simulink model "sf_test"  (R2020a)
settings: Solver=FixedStepDiscrete  StartTime=0.0  StopTime=10.0  RelTol=1e-3
settings Model: Creator=김진성  LastModifiedBy=노호진
settings OptimizationCC: DefaultParameterBehavior=Inlined  EnhancedBackFolding=on  PassReuseOutputArgsAs=Individual arguments  OptimizeBlockOrder=speed  DifferentSizesBufferReuse=on  OptimizationCustomize=off  EfficientTunableParamExpr=on
settings DebuggingCC: ParameterTunabilityLossMsg=error
settings HardwareCC: ProdBitPerPointer=32  ProdBitPerSizeT=32  ProdBitPerPtrDiffT=32  ProdLargestAtomicInteger=Long  ProdLargestAtomicFloat=Double  ProdWordSize=32  ProdHWDeviceType=ARM Compatible->ARM Cortex
settings SFSimCC: MATLABDynamicMemAlloc=off
settings RTWCC: SystemTargetFile=ert.tlc  GenCodeOnly=on  TemplateMakefile=ert_default_tmf  GenerateReport=on  IncludeHyperlinkInReport=on  LaunchReport=on  GenerateTraceInfo=on  GenerateTraceReport=on  GenerateTraceReportSl=on  GenerateTraceReportSf=on  GenerateTraceReportEml=on  GenerateCodeMetricsReport=on  GenerateCodeReplacementReport=on
settings CodeAppCC: ForceParamTrailComments=on  IgnoreCustomStorageClasses=off  OperatorAnnotations=on  SimulinkDataObjDesc=on  SFDataObjDesc=on  InsertBlockDesc=on  StateflowObjectComments=on
settings ERTTargetCC: TargetLangStandard=C99 (ISO)  GenerateSampleERTMain=on  MultiInstanceERTCode=on  CodeInterfacePackaging=Reusable function  InlinedParameterPlacement=NonHierarchical  ERTCustomFileTemplate=example_file_process.tlc

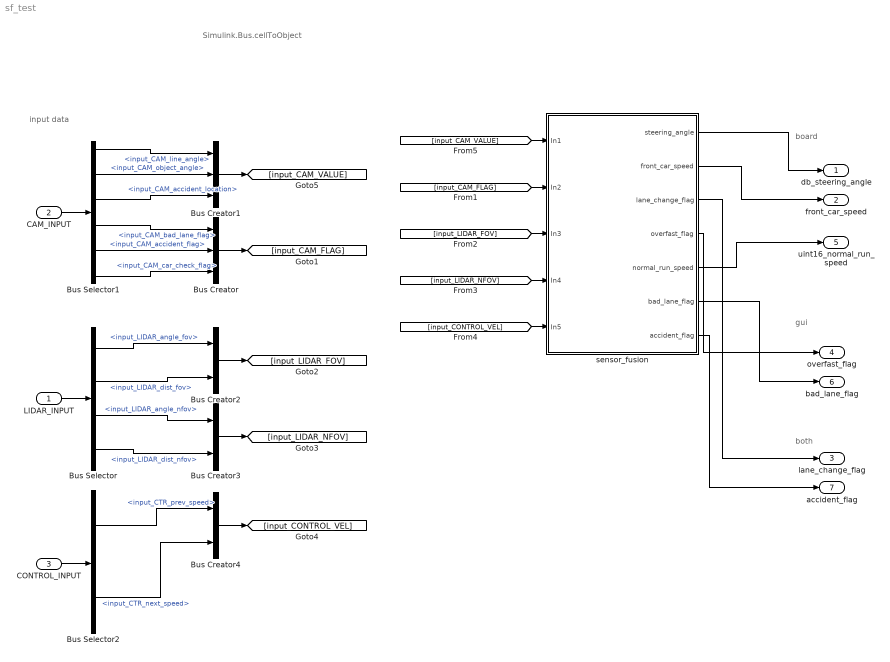
== system sf_test ==
  note: Simulink.Bus.cellToObject
  note: both
  note: gui
  note: board
  note: input data
  LIDAR_INPUT : Inport  OutDataTypeStr=Bus: LIDAR
  CAM_INPUT : Inport  Port=2  OutDataTypeStr=Bus: CAM
  CONTROL_INPUT : Inport  Port=3  OutDataTypeStr=Bus: CONTROL
  Bus Creator : BusCreator  Inputs=3
  Bus Creator1 : BusCreator  Inputs=3
  Bus Creator2 : BusCreator  Inputs=2
  Bus Creator3 : BusCreator  Inputs=2
  Bus Creator4 : BusCreator  Inputs=2
  Bus Selector : BusSelector  OutputSignals=input_LIDAR_angle_fov,input_LIDAR_dist_fov,input_LIDAR_angle_nfov,input_LIDAR_dist_nfov
  Bus Selector1 : BusSelector  OutputSignals=input_CAM_line_angle,input_CAM_object_angle,input_CAM_accident_location,input_CAM_bad_lane_flag,input_CAM_accident_flag,input_CAM_car_check_flag
  Bus Selector2 : BusSelector  OutputSignals=input_CTR_prev_speed,input_CTR_next_speed
  sensor_fusion : Subsystem  TreatAsAtomicUnit=on
      settings: RTWSystemCode=Nonreusable function  RTWFcnNameOpts=Use subsystem name
  db_steering_angle : Outport
  front_car_speed : Outport  Port=2
  lane_change_flag : Outport  Port=3
  overfast_flag : Outport  Port=4
  uint16_normal_run_speed : Outport  Port=5  OutDataTypeStr=uint16
  bad_lane_flag : Outport  Port=6
  accident_flag : Outport  Port=7
  wires:
  sensor_fusion/1(steering_angle) -> db_steering_angle/1
  sensor_fusion/3(lane_change_flag) -> lane_change_flag/1
  sensor_fusion/4(overfast_flag) -> overfast_flag/1
  sensor_fusion/5(normal_run_speed) -> uint16_normal_run_speed/1
  sensor_fusion/2(front_car_speed) -> front_car_speed/1
  sensor_fusion/6(bad_lane_flag) -> bad_lane_flag/1
  sensor_fusion/7(accident_flag) -> accident_flag/1
  LIDAR_INPUT/1 -> Bus Selector/1
  CAM_INPUT/1 -> Bus Selector1/1
  CONTROL_INPUT/1 -> Bus Selector2/1
  Bus Selector1/1 -> Bus Creator1/1  "<input_CAM_line_angle>"
  Bus Selector1/2 -> Bus Creator1/2  "<input_CAM_object_angle>"
  Bus Selector1/3 -> Bus Creator1/3  "<input_CAM_accident_location>"
  Bus Selector1/4 -> Bus Creator/1  "<input_CAM_bad_lane_flag>"
  Bus Selector1/5 -> Bus Creator/2  "<input_CAM_accident_flag>"
  Bus Selector1/6 -> Bus Creator/3  "<input_CAM_car_check_flag>"
  Bus Creator/1 -> [input_CAM_FLAG]
  Bus Creator1/1 -> [input_CAM_VALUE]
  Bus Selector/1 -> Bus Creator2/1  "<input_LIDAR_angle_fov>"
  Bus Selector/2 -> Bus Creator2/2  "<input_LIDAR_dist_fov>"
  Bus Selector/3 -> Bus Creator3/1  "<input_LIDAR_angle_nfov>"
  Bus Selector/4 -> Bus Creator3/2  "<input_LIDAR_dist_nfov>"
  Bus Creator2/1 -> [input_LIDAR_FOV]
  Bus Creator3/1 -> [input_LIDAR_NFOV]
  Bus Selector2/1 -> Bus Creator4/1  "<input_CTR_prev_speed>"
  Bus Selector2/2 -> Bus Creator4/2  "<input_CTR_next_speed>"
  Bus Creator4/1 -> [input_CONTROL_VEL]
  [input_CAM_VALUE] -> sensor_fusion/1(In1)
  [input_CAM_FLAG] -> sensor_fusion/2(In2)
  [input_LIDAR_FOV] -> sensor_fusion/3(In3)
  [input_LIDAR_NFOV] -> sensor_fusion/4(In4)
  [input_CONTROL_VEL] -> sensor_fusion/5(In5)

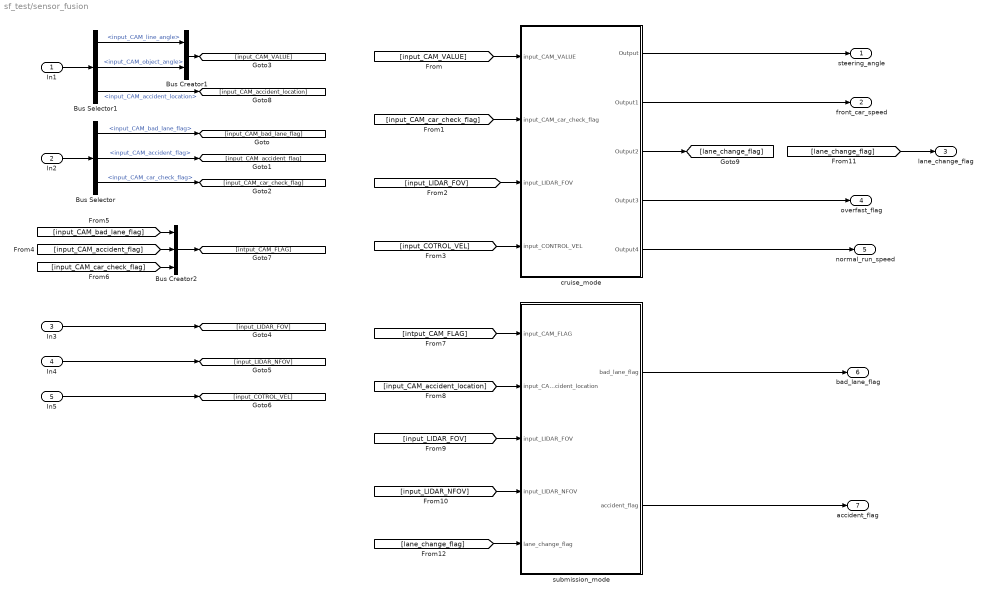
== system sf_test/sensor_fusion ==
  In1 : Inport
  In2 : Inport  Port=2
  In3 : Inport  Port=3
  In4 : Inport  Port=4
  In5 : Inport  Port=5
  Bus Creator1 : BusCreator  Inputs=2
  Bus Creator2 : BusCreator  Inputs=3
  Bus Selector : BusSelector  OutputSignals=input_CAM_bad_lane_flag,input_CAM_accident_flag,input_CAM_car_check_flag
  Bus Selector1 : BusSelector  OutputSignals=input_CAM_line_angle,input_CAM_object_angle,input_CAM_accident_location
  cruise_mode : Subsystem  TreatAsAtomicUnit=on
      settings: RTWSystemCode=Nonreusable function  RTWFcnNameOpts=Use subsystem name
  submission_mode : Subsystem  TreatAsAtomicUnit=on
      settings: RTWSystemCode=Nonreusable function  RTWFcnNameOpts=Use subsystem name
  steering_angle : Outport
  front_car_speed : Outport  Port=2
  lane_change_flag : Outport  Port=3
  overfast_flag : Outport  Port=4
  normal_run_speed : Outport  Port=5  OutDataTypeStr=uint16
  bad_lane_flag : Outport  Port=6
  accident_flag : Outport  Port=7
  wires:
  cruise_mode/1(Output) -> steering_angle/1
  cruise_mode/2(Output1) -> front_car_speed/1
  cruise_mode/4(Output3) -> overfast_flag/1
  cruise_mode/5(Output4) -> normal_run_speed/1
  submission_mode/1(bad_lane_flag) -> bad_lane_flag/1
  submission_mode/2(accident_flag) -> accident_flag/1
  Bus Selector/1 -> [input_CAM_bad_lane_flag]  "<input_CAM_bad_lane_flag>"
  Bus Selector/2 -> [input_CAM_accident_flag]  "<input_CAM_accident_flag>"
  Bus Selector/3 -> [input_CAM_car_check_flag]  "<input_CAM_car_check_flag>"
  In3/1 -> [input_LIDAR_FOV]
  In4/1 -> [input_LIDAR_NFOV]
  In5/1 -> [input_COTROL_VEL]
  [input_CAM_VALUE] -> cruise_mode/1(input_CAM_VALUE)
  [input_CAM_car_check_flag] -> cruise_mode/2(input_CAM_car_check_flag)
  [input_LIDAR_FOV] -> cruise_mode/3(input_LIDAR_FOV)
  [input_COTROL_VEL] -> cruise_mode/4(input_CONTROL_VEL)
  Bus Creator2/1 -> [intput_CAM_FLAG]
  [intput_CAM_FLAG] -> submission_mode/1(input_CAM_FLAG)
  In1/1 -> Bus Selector1/1
  Bus Selector1/1 -> Bus Creator1/1  "<input_CAM_line_angle>"
  Bus Selector1/2 -> Bus Creator1/2  "<input_CAM_object_angle>"
  Bus Selector1/3 -> [input_CAM_accident_location]  "<input_CAM_accident_location>"
  [input_CAM_accident_location] -> submission_mode/2(input_CAM_accident_location)
  [input_LIDAR_FOV] -> submission_mode/3(input_LIDAR_FOV)
  [input_LIDAR_NFOV] -> submission_mode/4(input_LIDAR_NFOV)
  Bus Creator1/1 -> [input_CAM_VALUE]
  [input_CAM_bad_lane_flag] -> Bus Creator2/1
  [input_CAM_accident_flag] -> Bus Creator2/2
  [input_CAM_car_check_flag] -> Bus Creator2/3
  In2/1 -> Bus Selector/1
  cruise_mode/3(Output2) -> [lane_change_flag]
  [lane_change_flag] -> lane_change_flag/1
  [lane_change_flag] -> submission_mode/5(lane_change_flag)

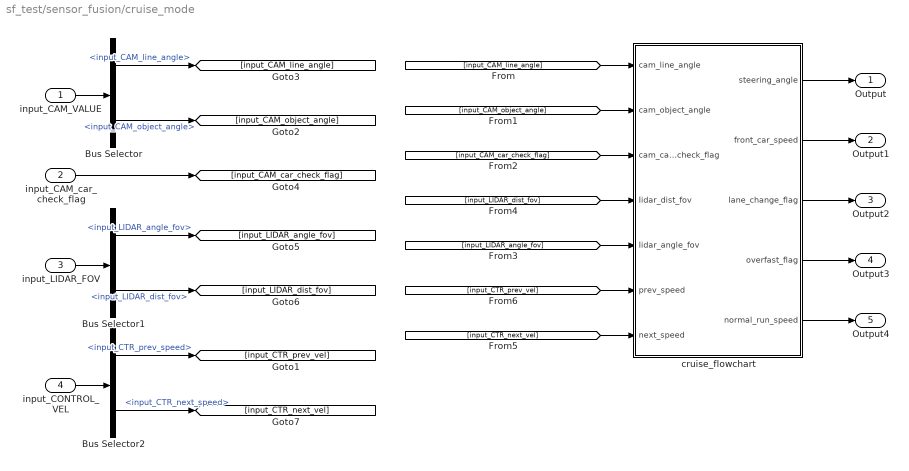
== system sf_test/sensor_fusion/cruise_mode ==
  input_CAM_VALUE : Inport
  input_CAM_car_check_flag : Inport  Port=2
  input_LIDAR_FOV : Inport  Port=3
  input_CONTROL_VEL : Inport  Port=4
  Bus Selector : BusSelector  OutputSignals=input_CAM_line_angle,input_CAM_object_angle
  Bus Selector1 : BusSelector  OutputSignals=input_LIDAR_angle_fov,input_LIDAR_dist_fov
  Bus Selector2 : BusSelector  OutputSignals=input_CTR_prev_speed,input_CTR_next_speed
  cruise_flowchart : Stateflow chart  TreatAsAtomicUnit=on
      settings: RTWSystemCode=Nonreusable function  RTWFcnNameOpts=Use subsystem name
  Output : Outport
  Output1 : Outport  Port=2
  Output2 : Outport  Port=3
  Output3 : Outport  Port=4
  Output4 : Outport  Port=5
  wires:
  [input_CAM_line_angle] -> cruise_flowchart/1(cam_line_angle)
  [input_CAM_object_angle] -> cruise_flowchart/2(cam_object_angle)
  [input_CAM_car_check_flag] -> cruise_flowchart/3(cam_car_check_flag)
  [input_LIDAR_angle_fov] -> cruise_flowchart/5(Iidar_angle_fov)
  cruise_flowchart/1(steering_angle) -> Output/1
  cruise_flowchart/2(front_car_speed) -> Output1/1
  [input_CTR_prev_vel] -> cruise_flowchart/6(prev_speed)
  [input_CTR_next_vel] -> cruise_flowchart/7(next_speed)
  cruise_flowchart/3(lane_change_flag) -> Output2/1
  cruise_flowchart/4(overfast_flag) -> Output3/1
  cruise_flowchart/5(normal_run_speed) -> Output4/1
  input_CAM_VALUE/1 -> Bus Selector/1
  Bus Selector/1 -> [input_CAM_line_angle]  "<input_CAM_line_angle>"
  Bus Selector/2 -> [input_CAM_object_angle]  "<input_CAM_object_angle>"
  input_CAM_car_check_flag/1 -> [input_CAM_car_check_flag]
  input_LIDAR_FOV/1 -> Bus Selector1/1
  Bus Selector1/1 -> [input_LIDAR_angle_fov]  "<input_LIDAR_angle_fov>"
  Bus Selector1/2 -> [input_LIDAR_dist_fov]  "<input_LIDAR_dist_fov>"
  [input_LIDAR_dist_fov] -> cruise_flowchart/4(Iidar_dist_fov)
  input_CONTROL_VEL/1 -> Bus Selector2/1
  Bus Selector2/1 -> [input_CTR_prev_vel]  "<input_CTR_prev_speed>"
  Bus Selector2/2 -> [input_CTR_next_vel]  "<input_CTR_next_speed>"

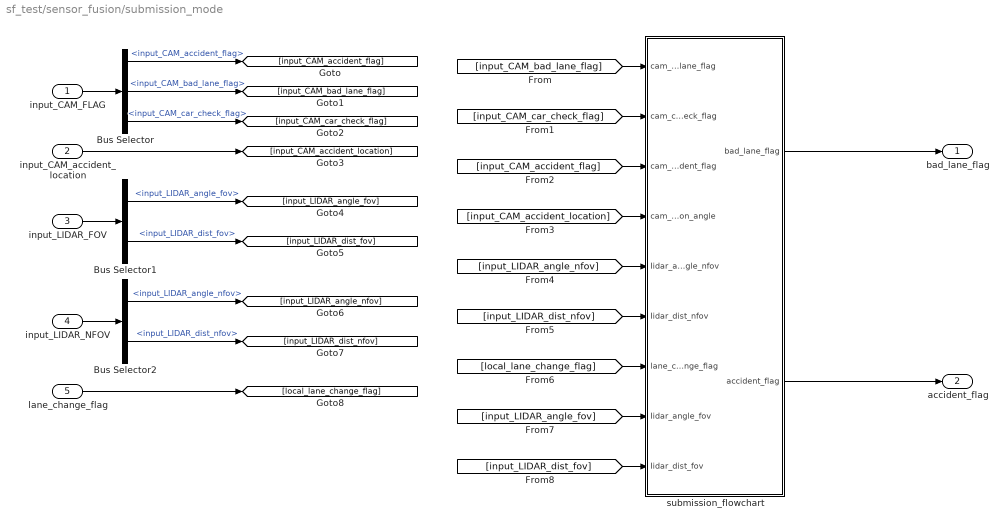
== system sf_test/sensor_fusion/submission_mode ==
  input_CAM_FLAG : Inport
  input_CAM_accident_location : Inport  Port=2
  input_LIDAR_FOV : Inport  Port=3
  input_LIDAR_NFOV : Inport  Port=4
  lane_change_flag : Inport  Port=5
  Bus Selector : BusSelector  OutputSignals=input_CAM_accident_flag,input_CAM_bad_lane_flag,input_CAM_car_check_flag
  Bus Selector1 : BusSelector  OutputSignals=input_LIDAR_angle_fov,input_LIDAR_dist_fov
  Bus Selector2 : BusSelector  OutputSignals=input_LIDAR_angle_nfov,input_LIDAR_dist_nfov
  submission_flowchart : Stateflow chart  TreatAsAtomicUnit=on
      settings: RTWSystemCode=Nonreusable function  RTWFcnNameOpts=Use subsystem name
  bad_lane_flag : Outport
  accident_flag : Outport  Port=2
  wires:
  [input_CAM_bad_lane_flag] -> submission_flowchart/1(cam_bad_lane_flag)
  [input_CAM_car_check_flag] -> submission_flowchart/2(cam_car_check_flag)
  [input_CAM_accident_flag] -> submission_flowchart/3(cam_accident_flag)
  [input_CAM_accident_location] -> submission_flowchart/4(cam_accident_location_angle)
  [input_LIDAR_angle_nfov] -> submission_flowchart/5(Iidar_angle_nfov)
  [input_LIDAR_dist_nfov] -> submission_flowchart/6(Iidar_dist_nfov)
  [local_lane_change_flag] -> submission_flowchart/7(lane_change_flag)
  [input_LIDAR_angle_fov] -> submission_flowchart/8(Iidar_angle_fov)
  submission_flowchart/1(bad_lane_flag) -> bad_lane_flag/1
  submission_flowchart/2(accident_flag) -> accident_flag/1
  input_CAM_FLAG/1 -> Bus Selector/1
  Bus Selector/1 -> [input_CAM_accident_flag]  "<input_CAM_accident_flag>"
  Bus Selector/2 -> [input_CAM_bad_lane_flag]  "<input_CAM_bad_lane_flag>"
  Bus Selector/3 -> [input_CAM_car_check_flag]  "<input_CAM_car_check_flag>"
  input_CAM_accident_location/1 -> [input_CAM_accident_location]
  input_LIDAR_FOV/1 -> Bus Selector1/1
  input_LIDAR_NFOV/1 -> Bus Selector2/1
  Bus Selector1/1 -> [input_LIDAR_angle_fov]  "<input_LIDAR_angle_fov>"
  Bus Selector1/2 -> [input_LIDAR_dist_fov]  "<input_LIDAR_dist_fov>"
  Bus Selector2/1 -> [input_LIDAR_angle_nfov]  "<input_LIDAR_angle_nfov>"
  Bus Selector2/2 -> [input_LIDAR_dist_nfov]  "<input_LIDAR_dist_nfov>"
  [input_LIDAR_dist_fov] -> submission_flowchart/9(Iidar_dist_fov)
  lane_change_flag/1 -> [local_lane_change_flag]

== stateflow chart sf_test/sensor_fusion/submission_mode/submission_flowchart ==
  state init_func
    state init
    state local_variable_init
      entry:
      local_lidar_dist_nfov = Iidar_dist_nfov;
      local_lider_angle_nfov = Iidar_angle_nfov;
      local_lidar_angle_fov = Iidar_angle_fov;
      local_lidar_dist_fov = Iidar_dist_fov;
    (default) -> init
    init -> local_variable_init [order 1] : [cam_car_check_flag==1]
  state bad_lane_func
    entry:
    bad_lane_flag = 1;
  note: -input data -
      | cam_bad_lane_flag
      | cam_car_check_flag
      | cam_accident_flag
      |
      | cam_accident_location_angle
      |
      | Iidar_angle_nfov
      | Iidar_dist_nfov
      | Iidar_angle_fov
      | Iidar_dist_fov
      |
      | lane_change_flag
  note: -output data -
      |
      | bad_lane_flag
      | accident_flag
  state accident_func
    entry:
    local_accident_location_angle = cam_accident_location_angle;
    accident_flag = 1;
  state lane_change_func
    entry:
  note: locla_variable_init 내부에 로컬 라이다 데이터(fov,nfov) 관련 처리 흐름도 추가할 것
  (default) -> init_func
  init -> bad_lane_func [order 2] : [cam_bad_lane_flag==1]
  local_variable_init -> accident_func [order 1] : [cam_accident_flag==1]
  local_variable_init -> lane_change_func [order 2] : [lane_change_flag==1]
  data: cam_bad_lane_flag input; cam_car_check_flag input; cam_accident_flag input; cam_accident_location_angle input; Iidar_angle_nfov input; Iidar_dist_nfov input; lane_change_flag input; local_lidar_dist_nfov local; local_lider_angle_nfov local; local_accident_location_angle local; Iidar_angle_fov input; Iidar_dist_fov input; local_lidar_angle_fov local; local_lidar_dist_fov local; bad_lane_flag output; accident_flag output

== stateflow chart sf_test/sensor_fusion/cruise_mode/cruise_flowchart ==
  state run_decision
    state front_car_decision
      en:
      local_object_angle = cam_object_angle;
      local_line_angle = cam_line_angle;
      local_lidar_angle = lidar_angle_fov;
    state front_car_velo_decision
      en:
      local_dist = lidar_dist_fov;
      sampling_time = time;
      state velo_calculation
        sampling_time = time - sampling_time;
      (default) -> velo_calculation
    state normal_run
      en:
      steering_angle = cam_line_angle;
      normal_run_speed = 200;
    (default) -> (junction 75)
    (junction 75) -> front_car_decision [order 2]
    (junction 75) -> normal_run [order 1] : [cam_car_check_flag == 0]
    front_car_decision -> (junction 93)
    (junction 93) -> front_car_velo_decision [order 2]
    (junction 93) -> (junction 128) [order 1] : [abs(local_lidar_angle - local_object_angle) > 5]
    front_car_velo_decision -> (junction 128) : [velo_calculation == 0]
    (junction 128) -> normal_run
  note: - input data -
      |
      | cam_line_angle:조향 각
      | cam_object_angle
      | cam_car_check_flag
      | //cam_bad_lane_flag
      | //cam_accident_flag
      | //cam_accident_location_angle
      |
      | lidar_dist_fov
      | lidar_angle_fov
      |
      | //lidar_dist_nfov
      | //lidar_angle_nfov
      |
      | //prev_speed
      | //next_speed
      |
      | time
  note: - output data -
      |
      | steering_angle
      | front_car_speed
      | lane_change_flag
      | normal_run_speed
  (default) -> run_decision
  data: cam_line_angle input; cam_object_angle input; cam_car_check_flag input; Iidar_dist_fov input; Iidar_angle_fov input; steering_angle output; local_object_angle local; local_line_angle local; local_current_speed_avr local; front_car_speed output; local_dist_diff local; prev_speed input; next_speed input; lane_change_flag output; overfast_flag output; car_check local double; normal_run_speed output uint16; lidar_angle_fov local; lidar_dist_fov local; local_dist local; local_lidar_angle local
